simulink model "s_parcial"  (R2022b)
settings: Solver=VariableStepAuto  StartTime=0.0  StopTime=200  RelTol=1e-3
libraries: simulink x1
settings Model: Creator=sophy  LastModifiedBy=sophy

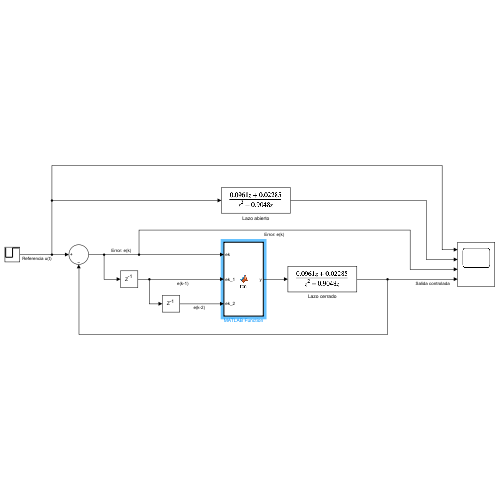
[thumbnail: Simulink's stored preview of the top-level diagram]
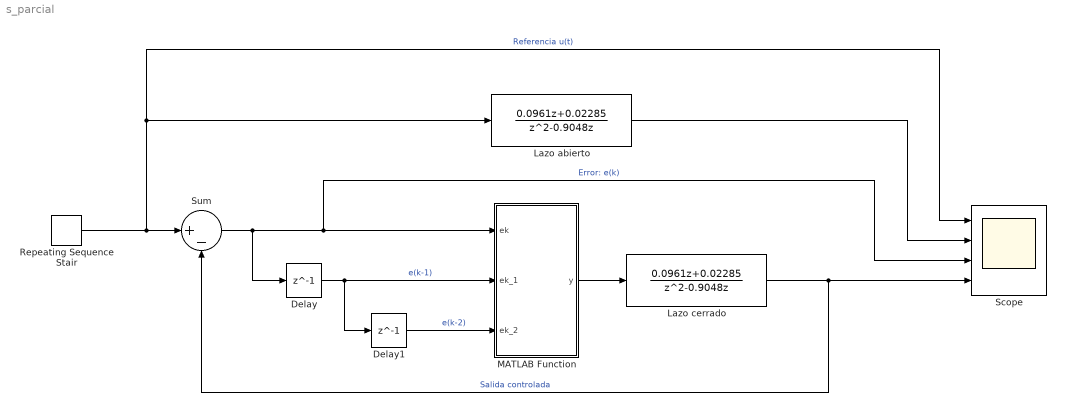
== system s_parcial ==
  Delay : Delay  DelayLength=1  SampleTime=2.5
  Delay1 : Delay  DelayLength=1  SampleTime=2.5
  Lazo abierto : DiscreteTransferFcn  Numerator=[0.0961 0.02285]  Denominator=[1 -0.9048 0]  SampleTime=2.5
  Lazo cerrado : DiscreteTransferFcn  Numerator=[0.0961 0.02285]  Denominator=[1 -0.9048 0]  SampleTime=2.5
  MATLAB Function : MATLAB Function  TreatAsAtomicUnit=on
  Repeating Sequence Stair : simulink/Sources/Repeating Sequence Stair  OutValues=[10 20].'  tsamp=100  OutMin=[]  OutMax=[]  OutDataTypeStr=double  OutputDataTypeScalingMode=double  OutDataType=fixdt(0,8)  ConRadixGroup=Best Precision: Vector-wise  OutScaling=2^-12
  Scope : Scope  NumInputPorts=4
  Sum : Sum  Inputs=|+-
  wires:
  Sum/1 -> Delay/1, Scope/3, MATLAB Function/1(ek)  "Error: e(k)"
  MATLAB Function/1(y) -> Lazo cerrado/1
  Lazo cerrado/1 -> Scope/4, Sum/2  "Salida controlada"
  Delay/1 -> Delay1/1, MATLAB Function/2(ek_1)  "e(k-1)"
  Delay1/1 -> MATLAB Function/3(ek_2)  "e(k-2)"
  Lazo abierto/1 -> Scope/2
  Repeating Sequence Stair/1 -> Scope/1, Lazo abierto/1, Sum/1  "Referencia u(t)"

== matlab function s_parcial/MATLAB Function ==
  data: ek input; y output; ek_1 input; ek_2 input
function y = fcn(ek, ek_1, ek_2)

persistent cant_neu_c1 cant_neu_c2 ...   % cant neuronas
    w_c1 w_c2 w_c3 ...                   % pesos sinapticos
    Yp_1 Yt_1 Yp_2 Yt_2 Yp_3 Yt_3 ...    % salidas
    n e1 e2 e3 ...                    % taza y retropropagacion

if isempty(w_c1)

    % Cantidad de neuronas por capa
    cant_neu_c1 = 6;
    cant_neu_c2 = 3;

    % Taza de aprendizaje
    n = 0.2;

    % Pesos sinapticos
    w_c1 = rand(cant_neu_c1, 3);             % Tres entradas: ek, ek_1 ek_2 
    w_c2 = rand(cant_neu_c2, cant_neu_c1);   % salida, entrada
    w_c3 = rand(1, cant_neu_c2);             % 1 salida

    % Error
    e1 = zeros(cant_neu_c1, 1);
    e2 = zeros(cant_neu_c2, 1);
    e3 = 0;

    % Salidas
    Yp_1 = zeros(cant_neu_c1, 1);
    Yt_1 = zeros(cant_neu_c1, 1);

    Yp_2 = zeros(cant_neu_c2, 1);
    Yt_2 = zeros(cant_neu_c2, 1);

    Yp_3 = 0;
    Yt_3 = 0;

end

% Normalizar
e = [ek, ek_1, ek_2]
e_max = max(e); 
e_min = min(e);

if e_max == e_min
    x = [ek, ek_1, ek_2]./e_max;
else
    x = (e - e_min) ./ (e_max - e_min);
end

%x = [ek, ek_1, ek_2]./15;


% Derivada sigmoide: ds = yT .* (1 - yT))

% Recorrer capas

% Capa oculta 1
Yp_1 = w_c1 * x'; 
Yt_1 = sigmoide(Yp_1);

% Capa oculta 2
Yp_2 = w_c2 * Yt_1;
Yt_2 = sigmoide(Yp_2);
    
% Capa final
Yp_3 = w_c3 * Yt_2;  
Yt_3 = sigmoide(Yp_3);
%Yt_3 = sigmoide(Yp_3)

% Error y retropropagacion
e3 = ek;
e2 = w_c3' * e3; 
e1 = w_c2' * e2;

% Actualización de pesos
w_c3 = w_c3 + n * e3 .* der_sigmoide(Yp_3) * Yt_2';
w_c2 = w_c2 + n * e2 .* der_sigmoide(Yp_2) * Yt_1';
w_c1 = w_c1 + n * e1 .* der_sigmoide(Yp_1) * x;

% Actualizo taza de aprendizaje
n = n+(0.0009*abs(ek));

% Salida
y = Yt_3*16.5

end

function yT = sigmoide(yP)
    yT = 1 ./ (1 + exp(-yP));
end

function ds = der_sigmoide(yP) % asi si uso Yp (como se define por derivada de sigmoide)
    % f*(1-f)
    sigmoid = 1 ./ (1 + exp(-yP));
    ds = sigmoid .* (1 - sigmoid);
end
